simulink model "controladores_movimiento"  (R2019a)
settings: Solver=VariableStepAuto  StartTime=0.0  StopTime=10.0  RelTol=1e-3
settings Model: Creator=Facundo  LastModifiedBy=Facundo

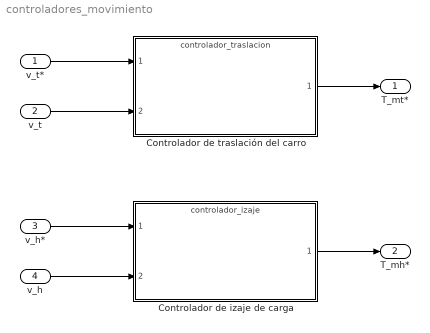
== system controladores_movimiento ==
  v_t* : Inport
  v_t : Inport  Port=2
  v_h* : Inport  Port=3
  v_h : Inport  Port=4
  Controlador de izaje de carga : ModelReference  ModelNameDialog=controlador_izaje.slx  SimulationMode=Normal  ModelReferenceVersion=1.6
  Controlador de traslación del carro : ModelReference  ModelNameDialog=controlador_traslacion.slx  SimulationMode=Normal  ModelReferenceVersion=1.5
  T_mt* : Outport
  T_mh* : Outport  Port=2
  wires:
  Controlador de traslación del carro/1 -> T_mt*/1
  Controlador de izaje de carga/1 -> T_mh*/1
  v_t*/1 -> Controlador de traslación del carro/1
  v_t/1 -> Controlador de traslación del carro/2
  v_h*/1 -> Controlador de izaje de carga/1
  v_h/1 -> Controlador de izaje de carga/2
